simulink model "MotorControlv7_dist_comp_sat_Exp"  (R2020b)
settings: Solver=ode4  StartTime=0.0  StopTime=0.1  FixedStep=0.0001  RelTol=1e-3
values from neighbouring files (symbols this model uses):
  b = 0,0    [motor_1stModel.m]
  J = 3.8e-7    (= 3.8e-07)    [motor_1stModel.m]
  K0 = R/Kt    (= 510.903426791)    [motor_1stModel.m]
  K1 = 1/K    [motor_1stModel.m]
  K2 = Tconst/K    [motor_1stModel.m]
  Ka = 24/1500    (= 0.016)    [motor_1stModel.m]
  Kc = 2048/2/3.141592    (= 325.949391264)    [motor_1stModel.m]
  Kd = 0    [motor_1stModel.m]
  Ke = 3.2086e-2    (= 0.032086)    [motor_1stModel.m]
  Ki = 0    [motor_1stModel.m]
  Kp = 1    [motor_1stModel.m]
  Kt = 3.21e-2    (= 0.0321)    [motor_1stModel.m]
  L = 0.0    (= 0)    [motor_1stModel.m]
  R = 16.4    [motor_1stModel.m]
libraries: pid_lib x1
settings Model: Creator=Owner  LastModifiedBy=Owner

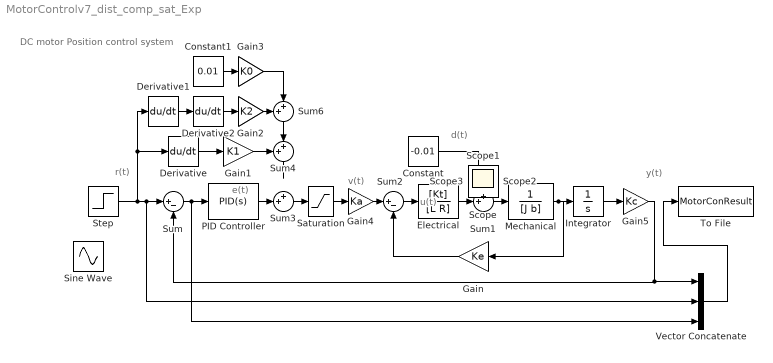
== system MotorControlv7_dist_comp_sat_Exp ==
  note: v(t)
  note: d(t)
  note: e(t)
  note: DC motor Position control system
  note: u(t)
  note: r(t)
  note: y(t)
  Constant : Constant  Value=-0.01
  Constant1 : Constant  Value=0.01
  Derivative : Derivative
  Derivative1 : Derivative
  Derivative2 : Derivative
  Electrical : TransferFcn  Numerator=[Kt]  Denominator=[L R]
  Gain : Gain  Gain=Ke
  Gain1 : Gain  Gain=K1
  Gain2 : Gain  Gain=K2
  Gain3 : Gain  Gain=K0
  Gain4 : Gain  Gain=Ka
  Gain5 : Gain  Gain=Kc
  Integrator : Integrator
  "Mechanical " : TransferFcn  Denominator=[J b]
  PID Controller : pid_lib/PID Controller  Controller=PID  Form=Parallel  TimeDomain=Continuous-time  UseExternalTs=off  SampleTime=-1  IntegratorMethod=Forward Euler  FilterMethod=Forward Euler  ControllerParametersSource=internal  P=Kp  I=Ki  D=Kd  UseFilter=on  N=1000  TunerSelectOption=Transfer Function Based (PID Tuner App)  InitialConditionSource=internal  InitialConditionForIntegrator=0  InitialConditionForFilter=0  DifferentiatorICPrevScaledInput=0  ExternalReset=none  TrackingMode=off  Kt=1  LimitOutput=off  SatLimitsSource=internal  UpperSaturationLimit=inf  LowerSaturationLimit=-inf  LinearizeAsGain=on  AntiWindupMode=none  Kb=1  POutMin=[]  POutMax=[]  IOutMin=[]  IOutMax=[]  DOutMin=[]  DOutMax=[]  NOutMin=[]  NOutMax=[]  SumOutMin=[]  SumOutMax=[]  SaturationOutMin=[]  SaturationOutMax=[]  PParamMin=[]  PParamMax=[]  IParamMin=[]  IParamMax=[]  DParamMin=[]  DParamMax=[]  NParamMin=[]  NParamMax=[]  KbParamMin=[]  KbParamMax=[]  KtParamMin=[]  KtParamMax=[]  KbOutMin=[]  KbOutMax=[]  KtOutMin=[]  KtOutMax=[]  IntegratorOutMin=[]  IntegratorOutMax=[]  FilterOutMin=[]  FilterOutMax=[]  SumI1OutMin=[]  SumI1OutMax=[]  SumI2OutMin=[]  SumI2OutMax=[]  SumI3OutMin=[]  SumI3OutMax=[]  SumI4OutMin=[]  SumI4OutMax=[]  SumDOutMin=[]  SumDOutMax=[]  DifferentiatorOutMin=[]  DifferentiatorOutMax=[]  FilterDiffOutCoefMin=[]  FilterDiffOutCoefMax=[]  ReciprocalOutMin=[]  ReciprocalOutMax=[]  SumDenOutMin=[]  SumDenOutMax=[]  SumNumOutMin=[]  SumNumOutMax=[]  DivideOutMin=[]  DivideOutMax=[]  UdiffTsProdOutMin=[]  UdiffTsProdOutMax=[]  NTsProdOutMin=[]  NTsProdOutMax=[]  UintegralTsProdOutMin=[]  UintegralTsProdOutMax=[]  UngainTsProdOutMin=[]  UngainTsProdOutMax=[]  IntegratorContinuousStateAttributes=''  IntegratorStateMustResolveToSignalObject=off  IntegratorRTWStateStorageClass=Auto  FilterContinuousStateAttributes=''  FilterStateMustResolveToSignalObject=off  FilterRTWStateStorageClass=Auto  ParallelPVariant=InternalParameters  IdealPVariant=Disabled  IVariant=InternalParameters  DVariant=InternalParameters  IntegratorVariant=Continuous  SatVariant=Disabled  AWVariant=Passthrough  PCopyVariant=Disabled  TRVariant=Disabled  FdbkBlocksVariant=Forward  IdealPFdbkVariant=Disabled  SatFdbkVariant=Disabled  DerivativeFilterVariant=ContFilter  NVariant=InternalParameters  NCopyVariant=Disabled  FilterICVariant=InternalICsFilter  IntegratorICVariant=InternalICs  ExternalResetVariant=Disabled  TRSumVariant=Passthrough  SumFdbkVariant=Disabled  SumVariant=Sum_PID  TsampFilterVariant=InternalTs  TsampNgainVariant=Passthrough  TsampIntegralVariant=Passthrough  ExternalSaturationOutDataTypeStr=Inherit: Same as second input
  Saturation : Saturate  UpperLimit=1500  LowerLimit=-1500
  Sine Wave : Sin  Bias=1  Frequency=(3.141592*2)*5  Phase=-3.141592/2  SampleTime=0
  Step : Step  Time=0  After=512  SampleTime=0
  Sum : Sum  Inputs=|+-
  Sum{1,3..4,6} (4 alike) : Sum  Inputs=++|
  Sum2 : Sum  Inputs=|+-
  To File : ToFile  Filename=MotorConResult
  Vector Concatenate : Concatenate  NumInputs=3
  Scope{,1..3} (4 alike) : Scope
  wires:
  Sum/1 -> Vector Concatenate/3, PID Controller/1
  PID Controller/1 -> Sum3/2
  Electrical/1 -> Sum1/2
  Sum1/1 -> "Mechanical "/1
  Constant/1 -> ?
  Gain5/1 -> Vector Concatenate/1, Sum/2
  "Mechanical "/1 -> Gain/1, Integrator/1
  Sum2/1 -> Electrical/1
  Gain/1 -> Sum2/2
  Saturation/1 -> Gain4/1
  Step/1 -> Vector Concatenate/2, Sum/1, Derivative1/1, Derivative/1
  Sum3/1 -> Saturation/1
  Derivative/1 -> Gain1/1
  Gain1/1 -> Sum4/1
  Sum4/1 -> ?
  Derivative1/1 -> Derivative2/1
  Derivative2/1 -> Gain2/1
  Gain2/1 -> Sum6/1
  Sum6/1 -> Sum4/2
  Constant1/1 -> Gain3/1
  Gain3/1 -> Sum6/2
  Vector Concatenate/1 -> To File/1
  Gain4/1 -> Sum2/1
  Integrator/1 -> Gain5/1
